simulink model "clutch_lockUp"  (R2020b)
settings: Solver=VariableStepAuto  StartTime=0.0  StopTime=10.0  RelTol=1e-3
values from neighbouring files (symbols this model uses):
  be = 2.0    [clutch_data.sldd]
  bv = 1.0    [clutch_data.sldd]
  Ie = 1.0    [clutch_data.sldd]
  Iv = 5.0    [clutch_data.sldd]
  muk = 1.0    [clutch_data.sldd]
  mus = 1.5    [clutch_data.sldd]
  R = 1.0    [clutch_data.sldd]
settings Model: DataDictionary=clutch_data.sldd  Creator=ADMIN  LastModifiedBy=ADMIN

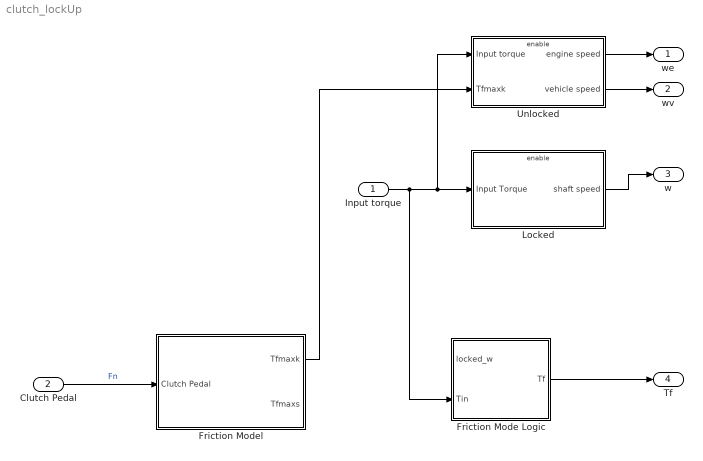
== system clutch_lockUp ==
  Input torque : Inport
  Clutch Pedal : Inport  Port=2
  Friction Mode Logic : Subsystem
  Friction Model : Subsystem
  Locked : Subsystem
  Unlocked : Subsystem
  we : Outport
  wv : Outport  Port=2
  w : Outport  Port=3
  Tf : Outport  Port=4
  wires:
  Input torque/1 -> Friction Mode Logic/2(Tin), Unlocked/1(Input torque), Locked/1(Input Torque)
  Unlocked/1(engine speed) -> we/1
  Unlocked/2(vehicle speed) -> wv/1
  Locked/1(shaft speed) -> w/1
  Clutch Pedal/1 -> Friction Model/1(Clutch Pedal)  "Fn"
  Friction Model/1(Tfmaxk) -> Unlocked/2(Tfmaxk)
  Friction Mode Logic/1(Tf) -> Tf/1

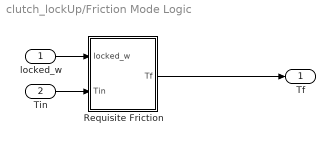
== system clutch_lockUp/Friction Mode Logic ==
  locked_w : Inport
  Tin : Inport  Port=2
  Requisite Friction : Subsystem
  Tf : Outport
  wires:
  Tin/1 -> Requisite Friction/2(Tin)
  locked_w/1 -> Requisite Friction/1(locked_w)
  Requisite Friction/1(Tf) -> Tf/1

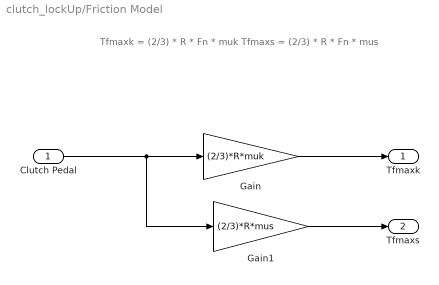
== system clutch_lockUp/Friction Model ==
  note: Tfmaxk = (2/3) * R * Fn * muk
      | Tfmaxs = (2/3) * R * Fn * mus
  Clutch Pedal : Inport
  Gain : Gain  Gain=(2/3)*R*muk
  Gain1 : Gain  Gain=(2/3)*R*mus
  Tfmaxk : Outport
  Tfmaxs : Outport  Port=2
  wires:
  Clutch Pedal/1 -> Gain1/1, Gain/1
  Gain/1 -> Tfmaxk/1
  Gain1/1 -> Tfmaxs/1

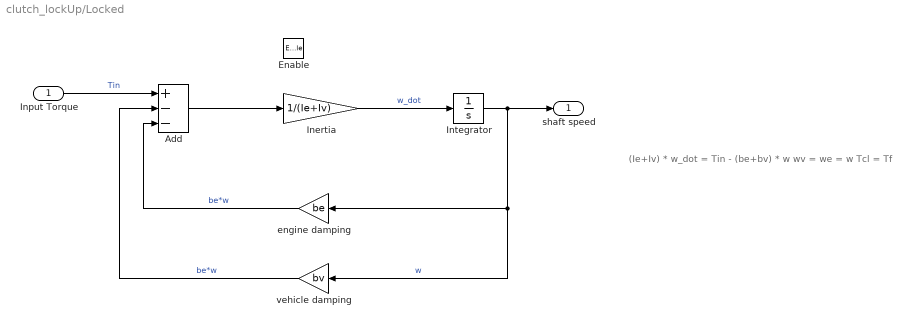
== system clutch_lockUp/Locked ==
  note: (Ie+Iv) * w_dot = Tin - (be+bv) * w
      | wv = we = w
      | Tcl = Tf
  Input Torque : Inport
  Enable : EnablePort
  Add : Sum  Inputs=+--
  Inertia : Gain  Gain=1/(Ie+Iv)
  Integrator : Integrator
  engine damping : Gain  Gain=be
  vehicle damping : Gain  Gain=bv
  shaft speed : Outport
  wires:
  Inertia/1 -> Integrator/1  "w_dot"
  Integrator/1 -> shaft speed/1, vehicle damping/1, engine damping/1  "w"
  Input Torque/1 -> Add/1  "Tin"
  engine damping/1 -> Add/3  "be*w"
  Add/1 -> Inertia/1
  vehicle damping/1 -> Add/2  "be*w"

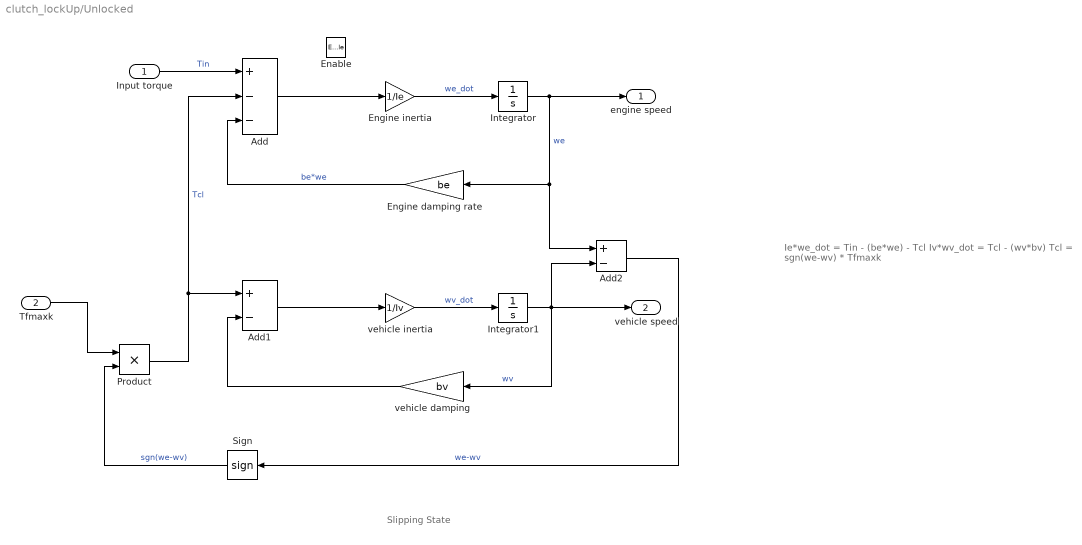
== system clutch_lockUp/Unlocked ==
  note: Slipping State
  note: Ie*we_dot = Tin - (be*we) - Tcl
      | Iv*wv_dot = Tcl - (wv*bv)
      | Tcl = sgn(we-wv) * Tfmaxk
  Input torque : Inport
  Tfmaxk : Inport  Port=2
  Enable : EnablePort
  Add : Sum  Inputs=+--
  Add1 : Sum  Inputs=+-
  Add2 : Sum  Inputs=+-
  Engine damping rate : Gain  Gain=be
  Engine inertia : Gain  Gain=1/Ie
  Integrator : Integrator
  Integrator1 : Integrator
  Product : Product
  Sign : Signum
  vehicle damping : Gain  Gain=bv
  vehicle inertia : Gain  Gain=1/Iv
  engine speed : Outport
  vehicle speed : Outport  Port=2
  wires:
  vehicle damping/1 -> Add1/2
  Product/1 -> Add1/1, Add/2  "Tcl"
  Sign/1 -> Product/2  "sgn(we-wv)"
  Tfmaxk/1 -> Product/1
  Engine damping rate/1 -> Add/3  "be*we"
  Input torque/1 -> Add/1  "Tin"
  Integrator1/1 -> vehicle speed/1, Add2/2, vehicle damping/1  "wv"
  Add2/1 -> Sign/1  "we-wv"
  Engine inertia/1 -> Integrator/1  "we_dot"
  Add/1 -> Engine inertia/1
  vehicle inertia/1 -> Integrator1/1  "wv_dot"
  Integrator/1 -> engine speed/1, Add2/1, Engine damping rate/1  "we"
  Add1/1 -> vehicle inertia/1

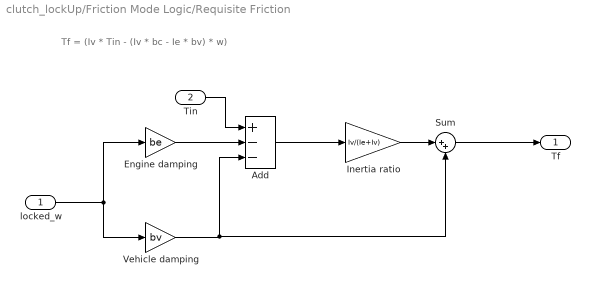
== system clutch_lockUp/Friction Mode Logic/Requisite Friction ==
  note: Tf = (Iv * Tin - (Iv * bc - Ie * bv) * w)
  locked_w : Inport
  Tin : Inport  Port=2
  Add : Sum  Inputs=+--
  Engine damping : Gain  Gain=be
  Inertia ratio : Gain  Gain=Iv/(Ie+Iv)
  Sum : Sum  Inputs=|++
  Vehicle damping : Gain  Gain=bv
  Tf : Outport
  wires:
  Inertia ratio/1 -> Sum/1
  locked_w/1 -> Vehicle damping/1, Engine damping/1
  Vehicle damping/1 -> Sum/2, Add/3
  Engine damping/1 -> Add/2
  Sum/1 -> Tf/1
  Tin/1 -> Add/1
  Add/1 -> Inertia ratio/1
